simulink library "G2ELib_V1"  (R2020b)
settings: Solver=VariableStepAuto  StartTime=0.0  StopTime=10.0  RelTol=1e-3
undefined symbols (not defined in the file or in its folder): ee_sli_rtmsupport, Filter, Filter_I_ini, Filter_V_ini, gcbh, GFM, GFM_L2, GFM_R2, Parameters_Ib, Parameters_Sb, Parameters_Un_dc, q_filter_wf, References_Q, References_Theta_Eg0, simlt, sps_rtmsupport, Vdc_loop
libraries: powerlib x48, simulink_extras x11, eeTransforms x10, pid_lib x8, spsSourcesModel x3, powerlib_meascontrol x3, spsVIMeasurementModel x3, spsFirstOrderFilterModel x3, spsSynchronousMachineModel x3, eeGeneralControl x2, eePowerMeasurement x1, sps3phSaturableTransformerModel x1
(part 4 of 5)

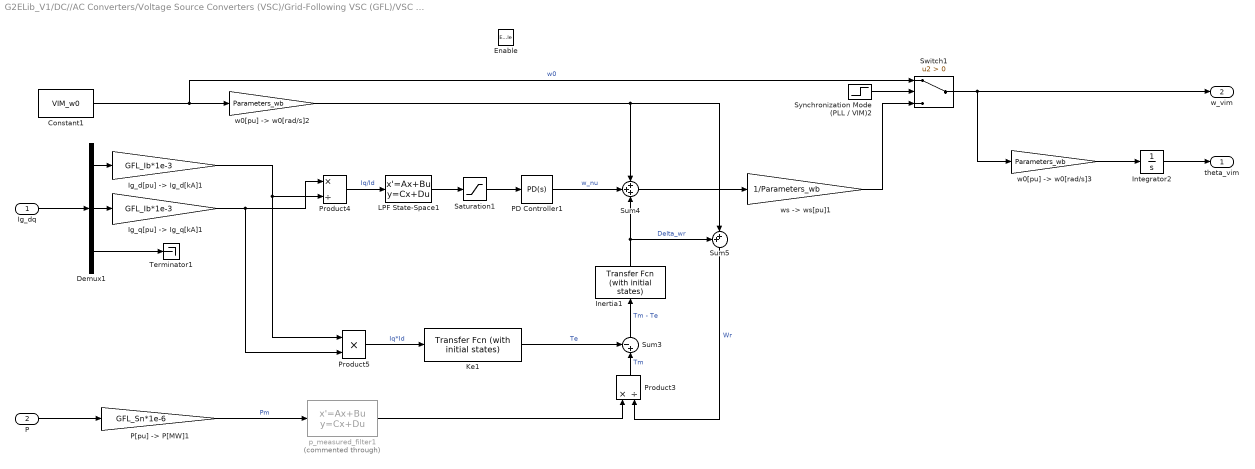
== system G2ELib_V1/DC//AC Converters/Voltage Source Converters (VSC)/Grid-Following VSC (GFL)/VSC - GFL - Ideal/VIM SU ==
  Ig_dq : Inport
  P : Inport  Port=2
  Enable : EnablePort
  Constant1 : Constant  Value=VIM_w0
  Demux1 : Demux  Outputs=3
      settings: DisplayOption=none
  "Ig_d[pu] -> Ig_d[kA]1" : Gain  Gain=GFL_Ib*1e-3
  "Ig_q[pu] -> Ig_q[kA]1" : Gain  Gain=GFL_Ib*1e-3
  Inertia1 : simulink_extras/Additional Linear/Transfer Fcn (with initial states)  N=1  D=[VIM_J VIM_D]  X0=VIM_Inertia_ini
  Integrator2 : Integrator  InitialCondition=GFL_theta
  Ke1 : simulink_extras/Additional Linear/Transfer Fcn (with initial states)  N=3/2.*VIM_Rr.*VIM_Lm.^2  D=[VIM_Lr.^2 , VIM_Rr.*VIM_Lr]  X0=VIM_Ke_ini
  LPF State-Space1 : StateSpace  A=-VIM_wc  C=VIM_wc  D=0  InitialCondition=VIM_wc_ini
  PD Controller1 : pid_lib/PID Controller  Controller=PD  Form=Parallel  TimeDomain=Continuous-time  UseExternalTs=off  SampleTime=-1  IntegratorMethod=Forward Euler  FilterMethod=Forward Euler  ControllerParametersSource=internal  P=VIM_Kp  I=0  D=VIM_Kd  UseFilter=on  N=VIM_Nd  TunerSelectOption=Transfer Function Based (PID Tuner App)  InitialConditionSource=internal  InitialConditionForIntegrator=0  InitialConditionForFilter=0  DifferentiatorICPrevScaledInput=0  ExternalReset=none  TrackingMode=off  Kt=1  LimitOutput=off  SatLimitsSource=internal  UpperSaturationLimit=inf  LowerSaturationLimit=-inf  LinearizeAsGain=on  AntiWindupMode=none  Kb=1  POutMin=[]  POutMax=[]  IOutMin=[]  IOutMax=[]  DOutMin=[]  DOutMax=[]  NOutMin=[]  NOutMax=[]  SumOutMin=[]  SumOutMax=[]  SaturationOutMin=[]  SaturationOutMax=[]  PParamMin=[]  PParamMax=[]  IParamMin=[]  IParamMax=[]  DParamMin=[]  DParamMax=[]  NParamMin=[]  NParamMax=[]  KbParamMin=[]  KbParamMax=[]  KtParamMin=[]  KtParamMax=[]  KbOutMin=[]  KbOutMax=[]  KtOutMin=[]  KtOutMax=[]  IntegratorOutMin=[]  IntegratorOutMax=[]  FilterOutMin=[]  FilterOutMax=[]  SumI1OutMin=[]  SumI1OutMax=[]  SumI2OutMin=[]  SumI2OutMax=[]  SumI3OutMin=[]  SumI3OutMax=[]  SumI4OutMin=[]  SumI4OutMax=[]  SumDOutMin=[]  SumDOutMax=[]  DifferentiatorOutMin=[]  DifferentiatorOutMax=[]  FilterDiffOutCoefMin=[]  FilterDiffOutCoefMax=[]  ReciprocalOutMin=[]  ReciprocalOutMax=[]  SumDenOutMin=[]  SumDenOutMax=[]  SumNumOutMin=[]  SumNumOutMax=[]  DivideOutMin=[]  DivideOutMax=[]  UdiffTsProdOutMin=[]  UdiffTsProdOutMax=[]  NTsProdOutMin=[]  NTsProdOutMax=[]  UintegralTsProdOutMin=[]  UintegralTsProdOutMax=[]  UngainTsProdOutMin=[]  UngainTsProdOutMax=[]  IntegratorContinuousStateAttributes=''  IntegratorStateMustResolveToSignalObject=off  IntegratorRTWStateStorageClass=Auto  FilterContinuousStateAttributes=''  FilterStateMustResolveToSignalObject=off  FilterRTWStateStorageClass=Auto  ParallelPVariant=InternalParameters  IdealPVariant=Disabled  IVariant=Disabled  DVariant=InternalParameters  IntegratorVariant=Disabled  SatVariant=Disabled  AWVariant=Disabled  PCopyVariant=Disabled  TRVariant=Disabled  FdbkBlocksVariant=Forward  IdealPFdbkVariant=Disabled  SatFdbkVariant=Disabled  DerivativeFilterVariant=ContFilter  NVariant=InternalParameters  NCopyVariant=Disabled  FilterICVariant=InternalICsFilter  IntegratorICVariant=Disabled  ExternalResetVariant=Disabled  TRSumVariant=Passthrough  SumFdbkVariant=Disabled  SumVariant=Sum_PD  TsampFilterVariant=InternalTs  TsampNgainVariant=Passthrough  TsampIntegralVariant=Disabled_SignalSpec  ExternalSaturationOutDataTypeStr=Inherit: Same as second input
  "P[pu] -> P[MW]1" : Gain  Gain=GFL_Sn*1e-6
  Product3 : Product  Inputs=*/
  Product4 : Product  Inputs=*/
  Product5 : Product
  Saturation1 : Saturate  UpperLimit=VIM_Iqd_sat  LowerLimit=-VIM_Iqd_sat
  Sum3 : Sum  Inputs=-+|
  Sum4 : Sum  Inputs=+++
  Sum5 : Sum  Inputs=++|
  Switch1 : Switch  Criteria=u2 > Threshold
  Synchronization Mode (PLL / VIM)2 : Step  Time=VIM_T_sync  Before=1  After=0  SampleTime=0
  Terminator1 : Terminator
  p_measured_filter1 : StateSpace  Commented=through  A=-q_filter_wf  C=q_filter_wf  D=0  InitialCondition=0
  "w0[pu] -> w0[rad/s]2" : Gain  Gain=Parameters_wb
  "w0[pu] -> w0[rad/s]3" : Gain  Gain=Parameters_wb
  "ws -> ws[pu]1" : Gain  Gain=1/Parameters_wb
  theta_vim : Outport
  w_vim : Outport  Port=2
  wires:
  p_measured_filter1/1 -> Product3/1
  Integrator2/1 -> theta_vim/1
  "w0[pu] -> w0[rad/s]3"/1 -> Integrator2/1
  Switch1/1 -> w_vim/1, "w0[pu] -> w0[rad/s]3"/1
  P/1 -> "P[pu] -> P[MW]1"/1
  Product4/1 -> LPF State-Space1/1  "Iq/Id"
  "Ig_q[pu] -> Ig_q[kA]1"/1 -> Product4/1, Product5/2
  Product3/1 -> Sum3/2  "Tm"
  PD Controller1/1 -> Sum4/2  "w_nu"
  Ke1/1 -> Sum3/1  "Te"
  Demux1/1 -> "Ig_d[pu] -> Ig_d[kA]1"/1
  Synchronization Mode (PLL / VIM)2/1 -> Switch1/2
  Sum4/1 -> "ws -> ws[pu]1"/1
  Demux1/2 -> "Ig_q[pu] -> Ig_q[kA]1"/1
  "Ig_d[pu] -> Ig_d[kA]1"/1 -> Product4/2, Product5/1
  Demux1/3 -> Terminator1/1
  Inertia1/1 -> Sum5/1, Sum4/3  "Delta_wr"
  Sum5/1 -> Product3/2  "Wr"
  LPF State-Space1/1 -> Saturation1/1
  Ig_dq/1 -> Demux1/1
  Product5/1 -> Ke1/1  "Iq*Id"
  Saturation1/1 -> PD Controller1/1
  "w0[pu] -> w0[rad/s]2"/1 -> Sum5/2, Sum4/1
  "P[pu] -> P[MW]1"/1 -> p_measured_filter1/1  "Pm"
  Sum3/1 -> Inertia1/1  "Tm - Te"
  "ws -> ws[pu]1"/1 -> Switch1/3
  Constant1/1 -> "w0[pu] -> w0[rad/s]2"/1, Switch1/1  "w0"

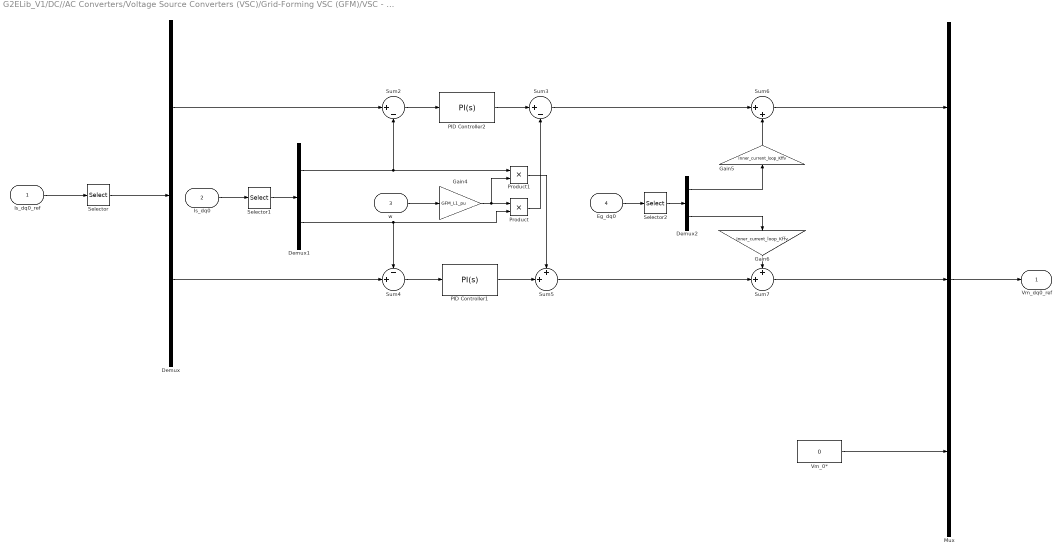
== system G2ELib_V1/DC//AC Converters/Voltage Source Converters (VSC)/Grid-Forming VSC (GFM)/VSC - GFM - Generic - Ideal/Current Loop ==
  Is_dq0_ref : Inport
  Is_dq0 : Inport  Port=2
  w : Inport  Port=3
  Eg_dq0 : Inport  Port=4
  Demux : Demux  Outputs=2
  Demux1 : Demux  Outputs=2
  Demux2 : Demux  Outputs=2
  Gain4 : Gain  Gain=GFM_L1_pu
  Gain5 : Gain  Gain=Inner_current_loop_Kffv
  Gain6 : Gain  Gain=Inner_current_loop_Kffv
  Mux : Mux  Inputs=3
  PID Controller1 : pid_lib/PID Controller  Controller=PI  Form=Parallel  TimeDomain=Continuous-time  UseExternalTs=off  SampleTime=-1  IntegratorMethod=Forward Euler  FilterMethod=Forward Euler  ControllerParametersSource=internal  P=Inner_current_loop_Kp  I=Inner_current_loop_Ki  D=0  UseFilter=on  N=100  TunerSelectOption=Transfer Function Based (PID Tuner App)  InitialConditionSource=internal  InitialConditionForIntegrator=Inner_current_loop_Int_ini_q  InitialConditionForFilter=0  DifferentiatorICPrevScaledInput=0  ExternalReset=none  TrackingMode=off  Kt=1  LimitOutput=off  SatLimitsSource=internal  UpperSaturationLimit=inf  LowerSaturationLimit=-inf  LinearizeAsGain=on  AntiWindupMode=none  Kb=1  POutMin=[]  POutMax=[]  IOutMin=[]  IOutMax=[]  DOutMin=[]  DOutMax=[]  NOutMin=[]  NOutMax=[]  SumOutMin=[]  SumOutMax=[]  SaturationOutMin=[]  SaturationOutMax=[]  PParamMin=[]  PParamMax=[]  IParamMin=[]  IParamMax=[]  DParamMin=[]  DParamMax=[]  NParamMin=[]  NParamMax=[]  KbParamMin=[]  KbParamMax=[]  KtParamMin=[]  KtParamMax=[]  KbOutMin=[]  KbOutMax=[]  KtOutMin=[]  KtOutMax=[]  IntegratorOutMin=[]  IntegratorOutMax=[]  FilterOutMin=[]  FilterOutMax=[]  SumI1OutMin=[]  SumI1OutMax=[]  SumI2OutMin=[]  SumI2OutMax=[]  SumI3OutMin=[]  SumI3OutMax=[]  SumI4OutMin=[]  SumI4OutMax=[]  SumDOutMin=[]  SumDOutMax=[]  DifferentiatorOutMin=[]  DifferentiatorOutMax=[]  FilterDiffOutCoefMin=[]  FilterDiffOutCoefMax=[]  ReciprocalOutMin=[]  ReciprocalOutMax=[]  SumDenOutMin=[]  SumDenOutMax=[]  SumNumOutMin=[]  SumNumOutMax=[]  DivideOutMin=[]  DivideOutMax=[]  UdiffTsProdOutMin=[]  UdiffTsProdOutMax=[]  NTsProdOutMin=[]  NTsProdOutMax=[]  UintegralTsProdOutMin=[]  UintegralTsProdOutMax=[]  UngainTsProdOutMin=[]  UngainTsProdOutMax=[]  IntegratorContinuousStateAttributes=''  IntegratorStateMustResolveToSignalObject=off  IntegratorRTWStateStorageClass=Auto  FilterContinuousStateAttributes=''  FilterStateMustResolveToSignalObject=off  FilterRTWStateStorageClass=Auto  ParallelPVariant=InternalParameters  IdealPVariant=Disabled  IVariant=InternalParameters  DVariant=Disabled  IntegratorVariant=Continuous  SatVariant=Disabled  AWVariant=Passthrough  PCopyVariant=Disabled  TRVariant=Disabled  FdbkBlocksVariant=Forward  IdealPFdbkVariant=Disabled  SatFdbkVariant=Disabled  DerivativeFilterVariant=Disabled  NVariant=Disabled  NCopyVariant=Disabled_SignalSpec  FilterICVariant=Disabled  IntegratorICVariant=InternalICs  ExternalResetVariant=Disabled  TRSumVariant=Passthrough  SumFdbkVariant=Disabled  SumVariant=Sum_PI  TsampFilterVariant=InternalTs  TsampNgainVariant=Passthrough  TsampIntegralVariant=Passthrough  ExternalSaturationOutDataTypeStr=Inherit: Same as second input
  PID Controller2 : pid_lib/PID Controller  Controller=PI  Form=Parallel  TimeDomain=Continuous-time  UseExternalTs=off  SampleTime=-1  IntegratorMethod=Forward Euler  FilterMethod=Forward Euler  ControllerParametersSource=internal  P=Inner_current_loop_Kp  I=Inner_current_loop_Ki  D=0  UseFilter=on  N=100  TunerSelectOption=Transfer Function Based (PID Tuner App)  InitialConditionSource=internal  InitialConditionForIntegrator=Inner_current_loop_Int_ini_d  InitialConditionForFilter=0  DifferentiatorICPrevScaledInput=0  ExternalReset=none  TrackingMode=off  Kt=1  LimitOutput=off  SatLimitsSource=internal  UpperSaturationLimit=inf  LowerSaturationLimit=-inf  LinearizeAsGain=on  AntiWindupMode=none  Kb=1  POutMin=[]  POutMax=[]  IOutMin=[]  IOutMax=[]  DOutMin=[]  DOutMax=[]  NOutMin=[]  NOutMax=[]  SumOutMin=[]  SumOutMax=[]  SaturationOutMin=[]  SaturationOutMax=[]  PParamMin=[]  PParamMax=[]  IParamMin=[]  IParamMax=[]  DParamMin=[]  DParamMax=[]  NParamMin=[]  NParamMax=[]  KbParamMin=[]  KbParamMax=[]  KtParamMin=[]  KtParamMax=[]  KbOutMin=[]  KbOutMax=[]  KtOutMin=[]  KtOutMax=[]  IntegratorOutMin=[]  IntegratorOutMax=[]  FilterOutMin=[]  FilterOutMax=[]  SumI1OutMin=[]  SumI1OutMax=[]  SumI2OutMin=[]  SumI2OutMax=[]  SumI3OutMin=[]  SumI3OutMax=[]  SumI4OutMin=[]  SumI4OutMax=[]  SumDOutMin=[]  SumDOutMax=[]  DifferentiatorOutMin=[]  DifferentiatorOutMax=[]  FilterDiffOutCoefMin=[]  FilterDiffOutCoefMax=[]  ReciprocalOutMin=[]  ReciprocalOutMax=[]  SumDenOutMin=[]  SumDenOutMax=[]  SumNumOutMin=[]  SumNumOutMax=[]  DivideOutMin=[]  DivideOutMax=[]  UdiffTsProdOutMin=[]  UdiffTsProdOutMax=[]  NTsProdOutMin=[]  NTsProdOutMax=[]  UintegralTsProdOutMin=[]  UintegralTsProdOutMax=[]  UngainTsProdOutMin=[]  UngainTsProdOutMax=[]  IntegratorContinuousStateAttributes=''  IntegratorStateMustResolveToSignalObject=off  IntegratorRTWStateStorageClass=Auto  FilterContinuousStateAttributes=''  FilterStateMustResolveToSignalObject=off  FilterRTWStateStorageClass=Auto  ParallelPVariant=InternalParameters  IdealPVariant=Disabled  IVariant=InternalParameters  DVariant=Disabled  IntegratorVariant=Continuous  SatVariant=Disabled  AWVariant=Passthrough  PCopyVariant=Disabled  TRVariant=Disabled  FdbkBlocksVariant=Forward  IdealPFdbkVariant=Disabled  SatFdbkVariant=Disabled  DerivativeFilterVariant=Disabled  NVariant=Disabled  NCopyVariant=Disabled_SignalSpec  FilterICVariant=Disabled  IntegratorICVariant=InternalICs  ExternalResetVariant=Disabled  TRSumVariant=Passthrough  SumFdbkVariant=Disabled  SumVariant=Sum_PI  TsampFilterVariant=InternalTs  TsampNgainVariant=Passthrough  TsampIntegralVariant=Passthrough  ExternalSaturationOutDataTypeStr=Inherit: Same as second input
  Product : Product
  Product1 : Product
  Selector : Selector  InputPortWidth=3  IndexOptions=Index vector (dialog)  Indices=[1 2]  OutputSizes=1
  Selector1 : Selector  InputPortWidth=3  IndexOptions=Index vector (dialog)  Indices=[1 2]  OutputSizes=1
  Selector2 : Selector  InputPortWidth=3  IndexOptions=Index vector (dialog)  Indices=[1 2]  OutputSizes=1
  Sum2 : Sum  Inputs=|+-
  Sum3 : Sum  Inputs=|+-
  Sum4 : Sum  Inputs=-+|
  Sum5 : Sum  Inputs=++|
  Sum6 : Sum  Inputs=|++
  Sum7 : Sum  Inputs=++|
  Vm_0* : Constant  Value=0
  Vm_dq0_ref : Outport
  wires:
  Demux1/1 -> Sum2/2, Product1/1
  Demux2/2 -> Gain6/1
  Demux2/1 -> Gain5/1
  Demux1/2 -> Sum4/1, Product/2
  PID Controller2/1 -> Sum3/1
  Selector/1 -> Demux/1
  Sum3/1 -> Sum6/1
  Gain5/1 -> Sum6/2
  Demux/1 -> Sum2/1
  PID Controller1/1 -> Sum5/2
  Gain4/1 -> Product1/2, Product/1
  Product/1 -> Sum3/2
  Selector1/1 -> Demux1/1
  w/1 -> Gain4/1
  Selector2/1 -> Demux2/1
  Vm_0*/1 -> Mux/3
  Is_dq0/1 -> Selector1/1
  Mux/1 -> Vm_dq0_ref/1
  Gain6/1 -> Sum7/1
  Sum2/1 -> PID Controller2/1
  Eg_dq0/1 -> Selector2/1
  Sum5/1 -> Sum7/2
  Sum4/1 -> PID Controller1/1
  Is_dq0_ref/1 -> Selector/1
  Product1/1 -> Sum5/1
  Demux/2 -> Sum4/2
  Sum6/1 -> Mux/1
  Sum7/1 -> Mux/2

== system G2ELib_V1/DC//AC Converters/Voltage Source Converters (VSC)/Grid-Forming VSC (GFM)/VSC - GFM - Generic - Ideal/DC Voltage Control  ==
  Vdc : Inport
  Vdc_ref : Inport  Port=2
  P_set : Inport  Port=3
  Gain : Gain  Gain=Vdc_loop_Ki
  Gain1 : Gain  Gain=Vdc_loop_Kp
  Gain2 : Gain  Gain=Parameters_Sb/(Parameters_Un_dc)
  Gain3 : Gain  Gain=Vdc_loop_Kffi
  Integrator : Integrator
  Sum : Sum  Inputs=|-+
  Sum1 : Sum  Inputs=+++
  idc_ref : Outport
  wires:
  Gain3/1 -> Sum1/1
  Gain2/1 -> Gain3/1
  Sum/1 -> Gain1/1, Gain/1
  Gain/1 -> Integrator/1
  P_set/1 -> Gain2/1
  Vdc/1 -> Sum/1
  Integrator/1 -> Sum1/2
  Sum1/1 -> idc_ref/1
  Vdc_ref/1 -> Sum/2
  Gain1/1 -> Sum1/3

== system G2ELib_V1/DC//AC Converters/Voltage Source Converters (VSC)/Grid-Forming VSC (GFM)/VSC - GFM - Generic - Ideal/Damping Resistor ==
  Ig_dq0 : Inport
  Gain : Gain  Gain=Damping_resistor_Rv
  Gain1 : Gain  Gain=Damping_resistor_Enable
  Subsystem : Subsystem
  Sum : Sum  Inputs=|+-
  dE_DR_dq0 : Outport
  wires:
  Gain1/1 -> dE_DR_dq0/1
  Sum/1 -> Gain1/1
  Subsystem/1(Out1) -> Sum/1
  Gain/1 -> Subsystem/1(In1), Sum/2
  Ig_dq0/1 -> Gain/1

== system G2ELib_V1/DC//AC Converters/Voltage Source Converters (VSC)/Grid-Forming VSC (GFM)/VSC - GFM - Generic - Ideal/Filter ==
  Ground : powerlib/Elements/Ground  LConnTagsString=a
  Series RLC Branch10 : PMComponent  DialogController=POWERSYS.PowerSysDialog  LoadFcn=sps_rtmsupport('LoadFcn',gcbh);  StartFcn=sps_rtmsupport('StartFcn',gcbh);  StopFcn=sps_rtmsupport('StopFcn',gcbh);  PhysicalDomain=powersysdomain  LeftPortType=p1  RightPortType=p1  LConnTagsString=__new0  RConnTagsString=__new0  mask(Series RLC Branch){BranchType=C, Resistance=GFM.R1, Inductance=GFM.L1, SetiL0=on, InitialCurrent=Filter.I_ini(1)*GFM.Ib, Capacitance=GFM_C, Setx0=off, InitialVoltage=Filter_V_ini(2), Measurements=None}
      mask prompts: BranchType "Branch type:"; Resistance "Resistance (Ohms):"; Inductance "Inductance (H):"; SetiL0 "Set the initial inductor current"; InitialCurrent "Inductor initial current (A):"; Capacitance "Capacitance (F):"; Setx0 "Set the initial capacitor voltage"; InitialVoltage "Capacitor initial voltage (V):"
      mask help:
      | Implements a series branch of RLC elements.
      | Use the 'Branch type' parameter to add or remove elements from the branch.
      mask init:
      | [s1,s2,s3,s4,r1,r2,l1,l2,c1,c2,c3,c4] = powericon('Series RLC Branch',Resistance,Inductance,Capacitance,BranchType);
      | powericon('RLCCback',gcb)
      | power_initmask();
      settings: CopyFcn=sps_rtmsupport('CopyFcn',gcbh);  DeleteFcn=sps_rtmsupport('DeleteFcn',gcbh);  UndoDeleteFcn=sps_rtmsupport('UndoDeleteFcn',gcbh);  ModelCloseFcn=sps_rtmsupport('ModelCloseFcn',gcbh);  PreSaveFcn=sps_rtmsupport('PreSaveFcn',gcbh);  PostSaveFcn=sps_rtmsupport('PostSaveFcn',gcbh);  NameChangeFcn=sps_rtmsupport('NameChangeFcn',gcbh);  PreCopyFcn=sps_rtmsupport('PreCopyFcn',gcbh);  OpenFcn=sps_rtmsupport('OpenFcn',gcbh, [1 4 7 9]);  CloseFcn=sps_rtmsupport('CloseFcn',gcbh);  PreDeleteFcn=sps_rtmsupport('PreDeleteFcn',gcbh);
      mask Help: helpview(psbhelp);
      mask TypeOptions BranchType: RLC | R | L | C | RL | RC | LC | Open circuit
      mask Callback BranchType: powericon('RLCCback',gcb)
      mask Callback Resistance: powericon('RLCCback',gcb)
      mask Callback Inductance: powericon('RLCCback',gcb)
      mask Callback SetiL0: powericon('RLCCback',gcb)
      mask Callback Capacitance: powericon('RLCCback',gcb)
      mask Callback Setx0: powericon('RLCCback',gcb)
      mask TypeOptions Measurements: None | Branch voltage | Branch current | Branch voltage and current
      mask Display:
      | plot(s1,s2,s3,s4,r1,r2*1.5,l1,l2*1.5,c1,c2*1.5,c3,c4*1.5)
      | color('red')
      | port_label('LConn',1,'+')
  Series RLC Branch11 : PMComponent  DialogController=POWERSYS.PowerSysDialog  LoadFcn=sps_rtmsupport('LoadFcn',gcbh);  StartFcn=sps_rtmsupport('StartFcn',gcbh);  StopFcn=sps_rtmsupport('StopFcn',gcbh);  PhysicalDomain=powersysdomain  LeftPortType=p1  RightPortType=p1  LConnTagsString=__new0  RConnTagsString=__new0  mask(Series RLC Branch){BranchType=C, Resistance=GFM.R1, Inductance=GFM.L1, SetiL0=on, InitialCurrent=Filter.I_ini(1)*GFM.Ib, Capacitance=GFM_C, Setx0=off, InitialVoltage=Filter_V_ini(3), Measurements=None}
      mask prompts: BranchType "Branch type:"; Resistance "Resistance (Ohms):"; Inductance "Inductance (H):"; SetiL0 "Set the initial inductor current"; InitialCurrent "Inductor initial current (A):"; Capacitance "Capacitance (F):"; Setx0 "Set the initial capacitor voltage"; InitialVoltage "Capacitor initial voltage (V):"
      mask help:
      | Implements a series branch of RLC elements.
      | Use the 'Branch type' parameter to add or remove elements from the branch.
      mask init:
      | [s1,s2,s3,s4,r1,r2,l1,l2,c1,c2,c3,c4] = powericon('Series RLC Branch',Resistance,Inductance,Capacitance,BranchType);
      | powericon('RLCCback',gcb)
      | power_initmask();
      settings: CopyFcn=sps_rtmsupport('CopyFcn',gcbh);  DeleteFcn=sps_rtmsupport('DeleteFcn',gcbh);  UndoDeleteFcn=sps_rtmsupport('UndoDeleteFcn',gcbh);  ModelCloseFcn=sps_rtmsupport('ModelCloseFcn',gcbh);  PreSaveFcn=sps_rtmsupport('PreSaveFcn',gcbh);  PostSaveFcn=sps_rtmsupport('PostSaveFcn',gcbh);  NameChangeFcn=sps_rtmsupport('NameChangeFcn',gcbh);  PreCopyFcn=sps_rtmsupport('PreCopyFcn',gcbh);  OpenFcn=sps_rtmsupport('OpenFcn',gcbh, [1 4 7 9]);  CloseFcn=sps_rtmsupport('CloseFcn',gcbh);  PreDeleteFcn=sps_rtmsupport('PreDeleteFcn',gcbh);
      mask Help: helpview(psbhelp);
      mask TypeOptions BranchType: RLC | R | L | C | RL | RC | LC | Open circuit
      mask Callback BranchType: powericon('RLCCback',gcb)
      mask Callback Resistance: powericon('RLCCback',gcb)
      mask Callback Inductance: powericon('RLCCback',gcb)
      mask Callback SetiL0: powericon('RLCCback',gcb)
      mask Callback Capacitance: powericon('RLCCback',gcb)
      mask Callback Setx0: powericon('RLCCback',gcb)
      mask TypeOptions Measurements: None | Branch voltage | Branch current | Branch voltage and current
      mask Display:
      | plot(s1,s2,s3,s4,r1,r2*1.5,l1,l2*1.5,c1,c2*1.5,c3,c4*1.5)
      | color('red')
      | port_label('LConn',1,'+')
  Series RLC Branch6 : PMComponent  DialogController=POWERSYS.PowerSysDialog  LoadFcn=sps_rtmsupport('LoadFcn',gcbh);  StartFcn=sps_rtmsupport('StartFcn',gcbh);  StopFcn=sps_rtmsupport('StopFcn',gcbh);  PhysicalDomain=powersysdomain  LeftPortType=p1  RightPortType=p1  LConnTagsString=__new0  RConnTagsString=__new0  mask(Series RLC Branch){BranchType=RL, Resistance=GFM_R1, Inductance=GFM_L1, SetiL0=off, InitialCurrent=Filter_I_ini(1), Capacitance=1e-6, Setx0=off, InitialVoltage=0, Measurements=None}
      mask prompts: BranchType "Branch type:"; Resistance "Resistance (Ohms):"; Inductance "Inductance (H):"; SetiL0 "Set the initial inductor current"; InitialCurrent "Inductor initial current (A):"; Capacitance "Capacitance (F):"; Setx0 "Set the initial capacitor voltage"; InitialVoltage "Capacitor initial voltage (V):"
      mask help:
      | Implements a series branch of RLC elements.
      | Use the 'Branch type' parameter to add or remove elements from the branch.
      mask init:
      | [s1,s2,s3,s4,r1,r2,l1,l2,c1,c2,c3,c4] = powericon('Series RLC Branch',Resistance,Inductance,Capacitance,BranchType);
      | powericon('RLCCback',gcb)
      | power_initmask();
      settings: CopyFcn=sps_rtmsupport('CopyFcn',gcbh);  DeleteFcn=sps_rtmsupport('DeleteFcn',gcbh);  UndoDeleteFcn=sps_rtmsupport('UndoDeleteFcn',gcbh);  ModelCloseFcn=sps_rtmsupport('ModelCloseFcn',gcbh);  PreSaveFcn=sps_rtmsupport('PreSaveFcn',gcbh);  PostSaveFcn=sps_rtmsupport('PostSaveFcn',gcbh);  NameChangeFcn=sps_rtmsupport('NameChangeFcn',gcbh);  PreCopyFcn=sps_rtmsupport('PreCopyFcn',gcbh);  OpenFcn=sps_rtmsupport('OpenFcn',gcbh, [1 4 7 9]);  CloseFcn=sps_rtmsupport('CloseFcn',gcbh);  PreDeleteFcn=sps_rtmsupport('PreDeleteFcn',gcbh);
      mask Help: helpview(psbhelp);
      mask TypeOptions BranchType: RLC | R | L | C | RL | RC | LC | Open circuit
      mask Callback BranchType: powericon('RLCCback',gcb)
      mask Callback Resistance: powericon('RLCCback',gcb)
      mask Callback Inductance: powericon('RLCCback',gcb)
      mask Callback SetiL0: powericon('RLCCback',gcb)
      mask Callback Capacitance: powericon('RLCCback',gcb)
      mask Callback Setx0: powericon('RLCCback',gcb)
      mask TypeOptions Measurements: None | Branch voltage | Branch current | Branch voltage and current
      mask Display:
      | plot(s1,s2,s3,s4,r1,r2*1.5,l1,l2*1.5,c1,c2*1.5,c3,c4*1.5)
      | color('red')
      | port_label('LConn',1,'+')
  Series RLC Branch7 : PMComponent  DialogController=POWERSYS.PowerSysDialog  LoadFcn=sps_rtmsupport('LoadFcn',gcbh);  StartFcn=sps_rtmsupport('StartFcn',gcbh);  StopFcn=sps_rtmsupport('StopFcn',gcbh);  PhysicalDomain=powersysdomain  LeftPortType=p1  RightPortType=p1  LConnTagsString=__new0  RConnTagsString=__new0  mask(Series RLC Branch){BranchType=RL, Resistance=GFM.R1, Inductance=GFM.L1, SetiL0=off, InitialCurrent=Filter_I_ini(2), Capacitance=1e-6, Setx0=off, InitialVoltage=0, Measurements=None}
      mask prompts: BranchType "Branch type:"; Resistance "Resistance (Ohms):"; Inductance "Inductance (H):"; SetiL0 "Set the initial inductor current"; InitialCurrent "Inductor initial current (A):"; Capacitance "Capacitance (F):"; Setx0 "Set the initial capacitor voltage"; InitialVoltage "Capacitor initial voltage (V):"
      mask help:
      | Implements a series branch of RLC elements.
      | Use the 'Branch type' parameter to add or remove elements from the branch.
      mask init:
      | [s1,s2,s3,s4,r1,r2,l1,l2,c1,c2,c3,c4] = powericon('Series RLC Branch',Resistance,Inductance,Capacitance,BranchType);
      | powericon('RLCCback',gcb)
      | power_initmask();
      settings: CopyFcn=sps_rtmsupport('CopyFcn',gcbh);  DeleteFcn=sps_rtmsupport('DeleteFcn',gcbh);  UndoDeleteFcn=sps_rtmsupport('UndoDeleteFcn',gcbh);  ModelCloseFcn=sps_rtmsupport('ModelCloseFcn',gcbh);  PreSaveFcn=sps_rtmsupport('PreSaveFcn',gcbh);  PostSaveFcn=sps_rtmsupport('PostSaveFcn',gcbh);  NameChangeFcn=sps_rtmsupport('NameChangeFcn',gcbh);  PreCopyFcn=sps_rtmsupport('PreCopyFcn',gcbh);  OpenFcn=sps_rtmsupport('OpenFcn',gcbh, [1 4 7 9]);  CloseFcn=sps_rtmsupport('CloseFcn',gcbh);  PreDeleteFcn=sps_rtmsupport('PreDeleteFcn',gcbh);
      mask Help: helpview(psbhelp);
      mask TypeOptions BranchType: RLC | R | L | C | RL | RC | LC | Open circuit
      mask Callback BranchType: powericon('RLCCback',gcb)
      mask Callback Resistance: powericon('RLCCback',gcb)
      mask Callback Inductance: powericon('RLCCback',gcb)
      mask Callback SetiL0: powericon('RLCCback',gcb)
      mask Callback Capacitance: powericon('RLCCback',gcb)
      mask Callback Setx0: powericon('RLCCback',gcb)
      mask TypeOptions Measurements: None | Branch voltage | Branch current | Branch voltage and current
      mask Display:
      | plot(s1,s2,s3,s4,r1,r2*1.5,l1,l2*1.5,c1,c2*1.5,c3,c4*1.5)
      | color('red')
      | port_label('LConn',1,'+')
  Series RLC Branch8 : PMComponent  DialogController=POWERSYS.PowerSysDialog  LoadFcn=sps_rtmsupport('LoadFcn',gcbh);  StartFcn=sps_rtmsupport('StartFcn',gcbh);  StopFcn=sps_rtmsupport('StopFcn',gcbh);  PhysicalDomain=powersysdomain  LeftPortType=p1  RightPortType=p1  LConnTagsString=__new0  RConnTagsString=__new0  mask(Series RLC Branch){BranchType=RL, Resistance=GFM.R1, Inductance=GFM.L1, SetiL0=off, InitialCurrent=Filter_I_ini(3), Capacitance=1e-6, Setx0=off, InitialVoltage=0, Measurements=None}
      mask prompts: BranchType "Branch type:"; Resistance "Resistance (Ohms):"; Inductance "Inductance (H):"; SetiL0 "Set the initial inductor current"; InitialCurrent "Inductor initial current (A):"; Capacitance "Capacitance (F):"; Setx0 "Set the initial capacitor voltage"; InitialVoltage "Capacitor initial voltage (V):"
      mask help:
      | Implements a series branch of RLC elements.
      | Use the 'Branch type' parameter to add or remove elements from the branch.
      mask init:
      | [s1,s2,s3,s4,r1,r2,l1,l2,c1,c2,c3,c4] = powericon('Series RLC Branch',Resistance,Inductance,Capacitance,BranchType);
      | powericon('RLCCback',gcb)
      | power_initmask();
      settings: CopyFcn=sps_rtmsupport('CopyFcn',gcbh);  DeleteFcn=sps_rtmsupport('DeleteFcn',gcbh);  UndoDeleteFcn=sps_rtmsupport('UndoDeleteFcn',gcbh);  ModelCloseFcn=sps_rtmsupport('ModelCloseFcn',gcbh);  PreSaveFcn=sps_rtmsupport('PreSaveFcn',gcbh);  PostSaveFcn=sps_rtmsupport('PostSaveFcn',gcbh);  NameChangeFcn=sps_rtmsupport('NameChangeFcn',gcbh);  PreCopyFcn=sps_rtmsupport('PreCopyFcn',gcbh);  OpenFcn=sps_rtmsupport('OpenFcn',gcbh, [1 4 7 9]);  CloseFcn=sps_rtmsupport('CloseFcn',gcbh);  PreDeleteFcn=sps_rtmsupport('PreDeleteFcn',gcbh);
      mask Help: helpview(psbhelp);
      mask TypeOptions BranchType: RLC | R | L | C | RL | RC | LC | Open circuit
      mask Callback BranchType: powericon('RLCCback',gcb)
      mask Callback Resistance: powericon('RLCCback',gcb)
      mask Callback Inductance: powericon('RLCCback',gcb)
      mask Callback SetiL0: powericon('RLCCback',gcb)
      mask Callback Capacitance: powericon('RLCCback',gcb)
      mask Callback Setx0: powericon('RLCCback',gcb)
      mask TypeOptions Measurements: None | Branch voltage | Branch current | Branch voltage and current
      mask Display:
      | plot(s1,s2,s3,s4,r1,r2*1.5,l1,l2*1.5,c1,c2*1.5,c3,c4*1.5)
      | color('red')
      | port_label('LConn',1,'+')
  Series RLC Branch9 : PMComponent  DialogController=POWERSYS.PowerSysDialog  LoadFcn=sps_rtmsupport('LoadFcn',gcbh);  StartFcn=sps_rtmsupport('StartFcn',gcbh);  StopFcn=sps_rtmsupport('StopFcn',gcbh);  PhysicalDomain=powersysdomain  LeftPortType=p1  RightPortType=p1  LConnTagsString=__new0  RConnTagsString=__new0  mask(Series RLC Branch){BranchType=C, Resistance=GFM.R1, Inductance=GFM.L1, SetiL0=on, InitialCurrent=Filter.I_ini(1)*GFM.Ib, Capacitance=GFM_C, Setx0=off, InitialVoltage=Filter_V_ini(1), Measurements=None}
      mask prompts: BranchType "Branch type:"; Resistance "Resistance (Ohms):"; Inductance "Inductance (H):"; SetiL0 "Set the initial inductor current"; InitialCurrent "Inductor initial current (A):"; Capacitance "Capacitance (F):"; Setx0 "Set the initial capacitor voltage"; InitialVoltage "Capacitor initial voltage (V):"
      mask help:
      | Implements a series branch of RLC elements.
      | Use the 'Branch type' parameter to add or remove elements from the branch.
      mask init:
      | [s1,s2,s3,s4,r1,r2,l1,l2,c1,c2,c3,c4] = powericon('Series RLC Branch',Resistance,Inductance,Capacitance,BranchType);
      | powericon('RLCCback',gcb)
      | power_initmask();
      settings: CopyFcn=sps_rtmsupport('CopyFcn',gcbh);  DeleteFcn=sps_rtmsupport('DeleteFcn',gcbh);  UndoDeleteFcn=sps_rtmsupport('UndoDeleteFcn',gcbh);  ModelCloseFcn=sps_rtmsupport('ModelCloseFcn',gcbh);  PreSaveFcn=sps_rtmsupport('PreSaveFcn',gcbh);  PostSaveFcn=sps_rtmsupport('PostSaveFcn',gcbh);  NameChangeFcn=sps_rtmsupport('NameChangeFcn',gcbh);  PreCopyFcn=sps_rtmsupport('PreCopyFcn',gcbh);  OpenFcn=sps_rtmsupport('OpenFcn',gcbh, [1 4 7 9]);  CloseFcn=sps_rtmsupport('CloseFcn',gcbh);  PreDeleteFcn=sps_rtmsupport('PreDeleteFcn',gcbh);
      mask Help: helpview(psbhelp);
      mask TypeOptions BranchType: RLC | R | L | C | RL | RC | LC | Open circuit
      mask Callback BranchType: powericon('RLCCback',gcb)
      mask Callback Resistance: powericon('RLCCback',gcb)
      mask Callback Inductance: powericon('RLCCback',gcb)
      mask Callback SetiL0: powericon('RLCCback',gcb)
      mask Callback Capacitance: powericon('RLCCback',gcb)
      mask Callback Setx0: powericon('RLCCback',gcb)
      mask TypeOptions Measurements: None | Branch voltage | Branch current | Branch voltage and current
      mask Display:
      | plot(s1,s2,s3,s4,r1,r2*1.5,l1,l2*1.5,c1,c2*1.5,c3,c4*1.5)
      | color('red')
      | port_label('LConn',1,'+')
  A : PMIOPort  Side=Left
  a : PMIOPort  Port=2  Side=Right
  B : PMIOPort  Port=3  Side=Left
  b : PMIOPort  Port=4  Side=Right
  C : PMIOPort  Port=5  Side=Left
  c : PMIOPort  Port=6  Side=Right
  connections:
  Series RLC Branch6/RConn1 -- a/RConn1 -- Series RLC Branch9/LConn1
  Series RLC Branch7/RConn1 -- b/RConn1 -- Series RLC Branch10/LConn1
  Series RLC Branch8/RConn1 -- c/RConn1 -- Series RLC Branch11/LConn1
  Series RLC Branch9/RConn1 -- Ground/LConn1 -- Series RLC Branch11/RConn1 -- Series RLC Branch10/RConn1
  C/RConn1 -- Series RLC Branch8/LConn1
  B/RConn1 -- Series RLC Branch7/LConn1
  A/RConn1 -- Series RLC Branch6/LConn1

== system G2ELib_V1/DC//AC Converters/Voltage Source Converters (VSC)/Grid-Forming VSC (GFM)/VSC - GFM - Generic - Ideal/Matching SU (SI) ==
  Vdc : Inport
  Vdc_ref : Inport  Port=2
  Enable : EnablePort
  Constant : Constant
  Gain : Gain  Gain=Matching_K_theta
  Gain1 : Gain
  Gain2 : Gain  Gain=1/GFM_Ub_dc
  Gain3 : Gain  Gain=Parameters_wb
  Gain4 : Gain
  Integrator : Integrator  InitialCondition=GFM_Theta_Eg0
  State-Space (with initial outputs)1 : simulink_extras/Additional Linear/State-Space (with initial outputs)  A=-q_filter_wf  B=1  C=q_filter_wf  D=0  U0=0  Y0=GFM_Vdcref/GFM_Ub_dc
      settings: SourceProductBaseCode=SL
  Sum : Sum  Inputs=|+-
  Sum1 : Sum  Inputs=++|
  theta : Outport
  w : Outport  Port=2
  wires:
  Gain/1 -> Sum1/2
  Vdc/1 -> Gain2/1
  Constant/1 -> Sum1/1
  Vdc_ref/1 -> Gain1/1
  Sum1/1 -> Gain4/1, Gain3/1
  Sum/1 -> Gain/1
  Integrator/1 -> theta/1
  Gain3/1 -> Integrator/1
  Gain1/1 -> Sum/2
  Gain4/1 -> w/1
  Gain2/1 -> State-Space (with initial outputs)1/1
  State-Space (with initial outputs)1/1 -> Sum/1

== system G2ELib_V1/DC//AC Converters/Voltage Source Converters (VSC)/Grid-Forming VSC (GFM)/VSC - GFM - Generic - Ideal/P-f Droop SU (PU) ==
  P : Inport
  P_set : Inport  Port=2
  w_set : Inport  Port=3
  Enable : EnablePort
  Gain : Gain  Gain=Droop_mp
  Gain1 : Gain  Gain=Parameters_wb
  Integrator : Integrator  InitialCondition=GFM_theta
  State-Space (with initial outputs) : simulink_extras/Additional Linear/State-Space (with initial outputs)  Commented=through  A=-Droop_wc  B=1  C=Droop_wc  D=0  U0=0  Y0=0
      settings: SourceProductBaseCode=SL
  State-Space (with initial outputs)1 : simulink_extras/Additional Linear/State-Space (with initial outputs)  A=-q_filter_wf  B=1  C=q_filter_wf  D=0  U0=0  Y0=GFM_Pref
      settings: SourceProductBaseCode=SL
  Sum : Sum  Inputs=+-|
  Sum1 : Sum  Inputs=++|
  theta : Outport
  w : Outport  Port=2
  wires:
  P/1 -> State-Space (with initial outputs)1/1
  Integrator/1 -> theta/1
  Gain1/1 -> Integrator/1
  Sum1/1 -> w/1, Gain1/1
  w_set/1 -> Sum1/1
  Sum/1 -> Gain/1
  Gain/1 -> State-Space (with initial outputs)/1
  P_set/1 -> Sum/1
  State-Space (with initial outputs)/1 -> Sum1/2
  State-Space (with initial outputs)1/1 -> Sum/2

== system G2ELib_V1/DC//AC Converters/Voltage Source Converters (VSC)/Grid-Forming VSC (GFM)/VSC - GFM - Generic - Ideal/PI_dc_voltage controller ==
  In : Inport
  Gain21 : Gain  Gain=Vdc_loop.Ki
  Gain22 : Gain  Gain=Vdc_loop.Kp
  Integrator1 : Integrator
  Sum6 : Sum  Inputs=++|
  out : Outport
  wires:
  Gain22/1 -> Sum6/1
  Integrator1/1 -> Sum6/2
  Gain21/1 -> Integrator1/1
  Sum6/1 -> out/1
  In/1 -> Gain21/1, Gain22/1

== system G2ELib_V1/DC//AC Converters/Voltage Source Converters (VSC)/Grid-Forming VSC (GFM)/VSC - GFM - Generic - Ideal/PLL ==
  Eg_abc : Inport
  Enable : EnablePort
  Constant : Constant
  Constant1 : Constant  Value=0
  Demux5 : Demux  Outputs=3
  Gain1 : Gain  Gain=0.0382
  Gain2 : Gain  Gain=0.2293
  Gain4 : Gain  Gain=Parameters_wb
  Integrator1 : Integrator  InitialCondition=GFM_theta
  Integrator3 : Integrator
  Low-Pass Filter (Discrete or Continuous) : eeGeneralControl/Low-Pass Filter (Discrete or Continuous)  Commented=through  K=1  T=0.01  B=inf  A=-inf  init_option=Specify as parameter  x0=1  Ts=simlt.T_step
  Park Transform3 : eeTransforms/Park Transform  AxisAlignment=Q-axis  PowerInvariant=off
  Sum : Sum  Inputs=|+-
  Sum1 : Sum  Inputs=|++
  Sum7 : Sum  Inputs=|++
  Terminator3 : Terminator
  Terminator4 : Terminator
  Transport Delay6 : TransportDelay  DelayTime=simlt.T_step  InitialOutput=Eg0_dq0
  w : Outport
  theta : Outport  Port=2
  wires:
  Sum7/1 -> Gain4/1, Low-Pass Filter (Discrete or Continuous)/1
  Gain2/1 -> Integrator3/1
  Gain4/1 -> Integrator1/1
  Eg_abc/1 -> Park Transform3/1
  Gain1/1 -> Sum1/1
  Demux5/2 -> Sum/1
  Sum1/1 -> Sum7/1
  Sum/1 -> Gain2/1, Gain1/1
  Demux5/3 -> Terminator3/1
  Demux5/1 -> Terminator4/1
  Integrator1/1 -> theta/1, Park Transform3/2
  Constant/1 -> Sum7/2
  Transport Delay6/1 -> Demux5/1
  Park Transform3/1 -> Transport Delay6/1
  Integrator3/1 -> Sum1/2
  Low-Pass Filter (Discrete or Continuous)/1 -> w/1
  Constant1/1 -> Sum/2

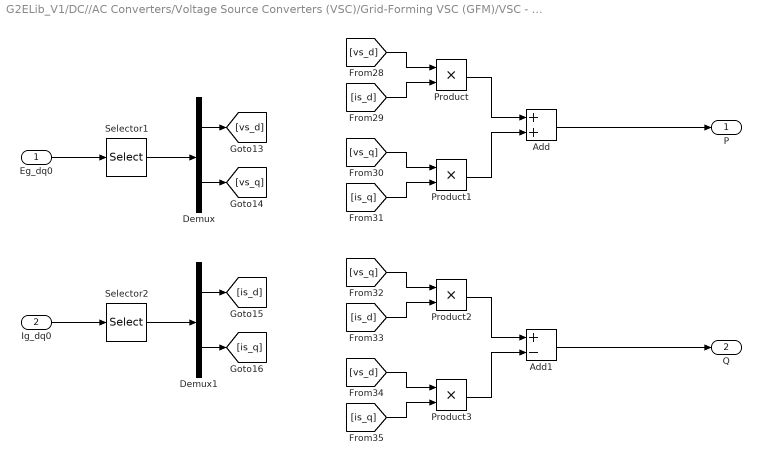
== system G2ELib_V1/DC//AC Converters/Voltage Source Converters (VSC)/Grid-Forming VSC (GFM)/VSC - GFM - Generic - Ideal/Power Measurement ==
  Eg_dq0 : Inport
  Ig_dq0 : Inport  Port=2
  Add : Sum
  Add1 : Sum  Inputs=+-
  Demux : Demux  Outputs=2
  Demux1 : Demux  Outputs=2
  Product{,1..3} (4 alike) : Product
  Selector1 : Selector  InputPortWidth=3  IndexOptions=Index vector (dialog)  Indices=[1 2]  OutputSizes=1
  Selector2 : Selector  InputPortWidth=3  IndexOptions=Index vector (dialog)  Indices=[1 2]  OutputSizes=1
  P : Outport
  Q : Outport  Port=2
  wires:
  Product/1 -> Add/1
  Product3/1 -> Add1/2
  Demux/1 -> [vs_d]
  [is_q] -> Product1/2
  [vs_q] -> Product1/1
  Selector2/1 -> Demux1/1
  [is_d] -> Product2/2
  [vs_d] -> Product3/1
  Product2/1 -> Add1/1
  Demux1/1 -> [is_d]
  [is_d] -> Product/2
  [vs_q] -> Product2/1
  Add1/1 -> Q/1
  Product1/1 -> Add/2
  [is_q] -> Product3/2
  Demux1/2 -> [is_q]
  Add/1 -> P/1
  Demux/2 -> [vs_q]
  [vs_d] -> Product/1
  Selector1/1 -> Demux/1
  Eg_dq0/1 -> Selector1/1
  Ig_dq0/1 -> Selector2/1

== system G2ELib_V1/DC//AC Converters/Voltage Source Converters (VSC)/Grid-Forming VSC (GFM)/VSC - GFM - Generic - Ideal/Q-V Droop MMU (PU) ==
  note: Generally only we set Eg_set_d only and Eg_set_q and Eg_set_0 equal zeros
  Q : Inport
  Q_set : Inport  Port=2
  Eg_set_dq0 : Inport  Port=3
  Enable : EnablePort
  Demux : Demux  Outputs=2
  Gain : Gain  Gain=Droop_nq
  Hypot : Math  Operator=hypot  SaturateOnIntegerOverflow=on
  Product : Product  Inputs=*/*
  Selector : Selector  InputPortWidth=3  IndexOptions=Index vector (dialog)  Indices=[1 2]  OutputSizes=1
  State-Space (with initial outputs)1 : simulink_extras/Additional Linear/State-Space (with initial outputs)  A=-q_filter_wf  B=1  C=q_filter_wf  D=0  U0=0  Y0=GFM_Qref
      settings: SourceProductBaseCode=SL
  Sum : Sum  Inputs=+-|
  Sum1 : Sum  Inputs=++|
  Eg_dq0_ref : Outport
  wires:
  Q/1 -> State-Space (with initial outputs)1/1
  Gain/1 -> Sum1/2
  Sum1/1 -> Product/1
  Q_set/1 -> Sum/1
  Eg_set_dq0/1 -> Product/3, Selector/1
  Selector/1 -> Demux/1
  Demux/2 -> Hypot/2
  Sum/1 -> Gain/1
  Demux/1 -> Hypot/1
  Hypot/1 -> Product/2, Sum1/1
  Product/1 -> Eg_dq0_ref/1
  State-Space (with initial outputs)1/1 -> Sum/2

== system G2ELib_V1/DC//AC Converters/Voltage Source Converters (VSC)/Grid-Forming VSC (GFM)/VSC - GFM - Generic - Ideal/Subsystem ==
  Vdq0 : Inport
  Add : Sum  Inputs=+++
  Demux : Demux  Outputs=3
  Product : Product
  Product1 : Product
  Product2 : Product
  Sqrt : Sqrt  SaturateOnIntegerOverflow=on
  Vrms : Outport
  wires:
  Add/1 -> Sqrt/1
  Product1/1 -> Add/2
  Sqrt/1 -> Vrms/1
  Vdq0/1 -> Demux/1
  Demux/2 -> Product1/1, Product1/2
  Product/1 -> Add/1
  Demux/1 -> Product/1, Product/2
  Demux/3 -> Product2/1, Product2/2
  Product2/1 -> Add/3

== system G2ELib_V1/DC//AC Converters/Voltage Source Converters (VSC)/Grid-Forming VSC (GFM)/VSC - GFM - Generic - Ideal/Subsystem1 ==
  Idq0 : Inport
  Add : Sum  Inputs=+++
  Demux : Demux  Outputs=3
  Product : Product
  Product1 : Product
  Product2 : Product
  Sqrt : Sqrt  SaturateOnIntegerOverflow=on
  Irms : Outport
  wires:
  Add/1 -> Sqrt/1
  Product1/1 -> Add/2
  Sqrt/1 -> Irms/1
  Idq0/1 -> Demux/1
  Demux/2 -> Product1/1, Product1/2
  Product/1 -> Add/1
  Demux/1 -> Product/1, Product/2
  Demux/3 -> Product2/1, Product2/2
  Product2/1 -> Add/3

== system G2ELib_V1/DC//AC Converters/Voltage Source Converters (VSC)/Grid-Forming VSC (GFM)/VSC - GFM - Generic - Ideal/Transient Virtual Impedance ==
  note: TVI triggering
  isd_mes_pu : Inport
  Demux : Demux  Outputs=2
  Demux1 : Demux  Outputs=2
      settings: DisplayOption=none
  Gain : Gain  Gain=TVI_K_RV
  Gain5 : Gain  Gain=TVI_Rho_XR
  Gain9 : Gain  Gain=TVI_Rho_XR
  Hypot : Math  Operator=hypot  SaturateOnIntegerOverflow=on
  I_tresh : Constant  Value=TVI_I_thresh_pu
  Mux2 : Mux  Inputs=3
  Selector1 : Selector  InputPortWidth=3  IndexOptions=Index vector (dialog)  Indices=[1 2]  OutputSizes=1
  Sum1 : Sum  Inputs=|+-
  Sum7 : Sum  Inputs=|+-
  Sum8 : Sum  Inputs=++|
  Switch2 : Switch
  dEg_0 : Constant  Value=0
  disabled : Constant  Value=0
  product{,1..3} (4 alike) : Product  InputSameDT=on  RndMeth=Zero  SaturateOnIntegerOverflow=on  OutDataTypeStr=Inherit: Same as first input
  dEg_dq0_VI : Outport
  wires:
  Gain9/1 -> Sum8/1
  I_tresh/1 -> Sum1/2
  Selector1/1 -> Switch2/1, Demux/1
  disabled/1 -> Switch2/3
  Switch2/1 -> Demux1/1
  Gain5/1 -> Sum7/2
  Sum1/1 -> Switch2/2, Gain/1
  dEg_0/1 -> Mux2/3
  product2/1 -> Sum8/2
  Demux/2 -> Hypot/2
  Demux/1 -> Hypot/1
  Demux1/2 -> product3/1, product2/1  "igq"
  isd_mes_pu/1 -> Selector1/1
  Demux1/1 -> product/2, product1/1  "Igd"
  Gain/1 -> product2/2, product1/2, product/1, product3/2
  Sum7/1 -> Mux2/1
  product3/1 -> Gain5/1
  product1/1 -> Sum7/1
  product/1 -> Gain9/1
  Sum8/1 -> Mux2/2
  Hypot/1 -> Sum1/1
  Mux2/1 -> dEg_dq0_VI/1

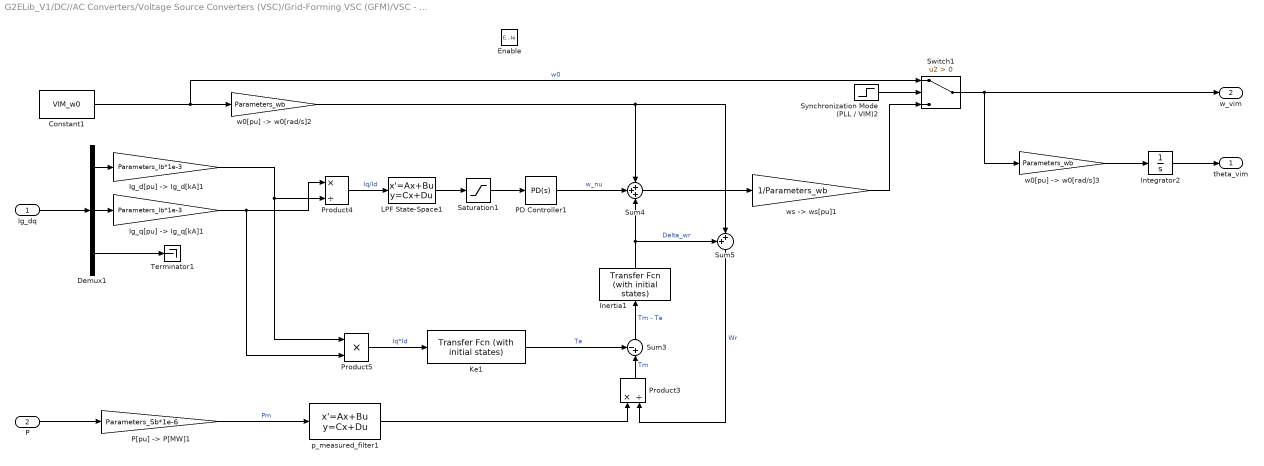
== system G2ELib_V1/DC//AC Converters/Voltage Source Converters (VSC)/Grid-Forming VSC (GFM)/VSC - GFM - Generic - Ideal/VIM SU ==
  Ig_dq : Inport
  P : Inport  Port=2
  Enable : EnablePort
  Constant1 : Constant  Value=VIM_w0
  Demux1 : Demux  Outputs=3
      settings: DisplayOption=none
  "Ig_d[pu] -> Ig_d[kA]1" : Gain  Gain=Parameters_Ib*1e-3
  "Ig_q[pu] -> Ig_q[kA]1" : Gain  Gain=Parameters_Ib*1e-3
  Inertia1 : simulink_extras/Additional Linear/Transfer Fcn (with initial states)  N=1  D=[VIM_J VIM_D]  X0=VIM_Inertia_ini
  Integrator2 : Integrator  InitialCondition=References_Theta_Eg0
  Ke1 : simulink_extras/Additional Linear/Transfer Fcn (with initial states)  N=3/2.*VIM_Rr.*VIM_Lm.^2  D=[VIM_Lr.^2 , VIM_Rr.*VIM_Lr]  X0=VIM_Ke_ini
  LPF State-Space1 : StateSpace  A=-VIM_wc  C=VIM_wc  D=0  InitialCondition=VIM_wc_ini
  PD Controller1 : pid_lib/PID Controller  Controller=PD  Form=Parallel  TimeDomain=Continuous-time  UseExternalTs=off  SampleTime=-1  IntegratorMethod=Forward Euler  FilterMethod=Forward Euler  ControllerParametersSource=internal  P=VIM_Kp  I=0  D=VIM_Kd  UseFilter=on  N=VIM_Nd  TunerSelectOption=Transfer Function Based (PID Tuner App)  InitialConditionSource=internal  InitialConditionForIntegrator=0  InitialConditionForFilter=0  DifferentiatorICPrevScaledInput=0  ExternalReset=none  TrackingMode=off  Kt=1  LimitOutput=off  SatLimitsSource=internal  UpperSaturationLimit=inf  LowerSaturationLimit=-inf  LinearizeAsGain=on  AntiWindupMode=none  Kb=1  POutMin=[]  POutMax=[]  IOutMin=[]  IOutMax=[]  DOutMin=[]  DOutMax=[]  NOutMin=[]  NOutMax=[]  SumOutMin=[]  SumOutMax=[]  SaturationOutMin=[]  SaturationOutMax=[]  PParamMin=[]  PParamMax=[]  IParamMin=[]  IParamMax=[]  DParamMin=[]  DParamMax=[]  NParamMin=[]  NParamMax=[]  KbParamMin=[]  KbParamMax=[]  KtParamMin=[]  KtParamMax=[]  KbOutMin=[]  KbOutMax=[]  KtOutMin=[]  KtOutMax=[]  IntegratorOutMin=[]  IntegratorOutMax=[]  FilterOutMin=[]  FilterOutMax=[]  SumI1OutMin=[]  SumI1OutMax=[]  SumI2OutMin=[]  SumI2OutMax=[]  SumI3OutMin=[]  SumI3OutMax=[]  SumI4OutMin=[]  SumI4OutMax=[]  SumDOutMin=[]  SumDOutMax=[]  DifferentiatorOutMin=[]  DifferentiatorOutMax=[]  FilterDiffOutCoefMin=[]  FilterDiffOutCoefMax=[]  ReciprocalOutMin=[]  ReciprocalOutMax=[]  SumDenOutMin=[]  SumDenOutMax=[]  SumNumOutMin=[]  SumNumOutMax=[]  DivideOutMin=[]  DivideOutMax=[]  UdiffTsProdOutMin=[]  UdiffTsProdOutMax=[]  NTsProdOutMin=[]  NTsProdOutMax=[]  UintegralTsProdOutMin=[]  UintegralTsProdOutMax=[]  UngainTsProdOutMin=[]  UngainTsProdOutMax=[]  IntegratorContinuousStateAttributes=''  IntegratorStateMustResolveToSignalObject=off  IntegratorRTWStateStorageClass=Auto  FilterContinuousStateAttributes=''  FilterStateMustResolveToSignalObject=off  FilterRTWStateStorageClass=Auto  ParallelPVariant=InternalParameters  IdealPVariant=Disabled  IVariant=Disabled  DVariant=InternalParameters  IntegratorVariant=Disabled  SatVariant=Disabled  AWVariant=Disabled  PCopyVariant=Disabled  TRVariant=Disabled  FdbkBlocksVariant=Forward  IdealPFdbkVariant=Disabled  SatFdbkVariant=Disabled  DerivativeFilterVariant=ContFilter  NVariant=InternalParameters  NCopyVariant=Disabled  FilterICVariant=InternalICsFilter  IntegratorICVariant=Disabled  ExternalResetVariant=Disabled  TRSumVariant=Passthrough  SumFdbkVariant=Disabled  SumVariant=Sum_PD  TsampFilterVariant=InternalTs  TsampNgainVariant=Passthrough  TsampIntegralVariant=Disabled_SignalSpec  ExternalSaturationOutDataTypeStr=Inherit: Same as second input
  "P[pu] -> P[MW]1" : Gain  Gain=Parameters_Sb*1e-6
  Product3 : Product  Inputs=*/
  Product4 : Product  Inputs=*/
  Product5 : Product
  Saturation1 : Saturate  UpperLimit=VIM_Iqd_sat  LowerLimit=-VIM_Iqd_sat
  Sum3 : Sum  Inputs=-+|
  Sum4 : Sum  Inputs=+++
  Sum5 : Sum  Inputs=++|
  Switch1 : Switch  Criteria=u2 > Threshold
  Synchronization Mode (PLL / VIM)2 : Step  Time=VIM_T_sync  Before=1  After=0  SampleTime=0
  Terminator1 : Terminator
  p_measured_filter1 : StateSpace  A=-q_filter_wf  C=q_filter_wf  D=0  InitialCondition=0
  "w0[pu] -> w0[rad/s]2" : Gain  Gain=Parameters_wb
  "w0[pu] -> w0[rad/s]3" : Gain  Gain=Parameters_wb
  "ws -> ws[pu]1" : Gain  Gain=1/Parameters_wb
  theta_vim : Outport
  w_vim : Outport  Port=2
  wires:
  p_measured_filter1/1 -> Product3/1
  Integrator2/1 -> theta_vim/1
  "w0[pu] -> w0[rad/s]3"/1 -> Integrator2/1
  Switch1/1 -> w_vim/1, "w0[pu] -> w0[rad/s]3"/1
  P/1 -> "P[pu] -> P[MW]1"/1
  Product4/1 -> LPF State-Space1/1  "Iq/Id"
  "Ig_q[pu] -> Ig_q[kA]1"/1 -> Product4/1, Product5/2
  Product3/1 -> Sum3/2  "Tm"
  PD Controller1/1 -> Sum4/2  "w_nu"
  Ke1/1 -> Sum3/1  "Te"
  Demux1/1 -> "Ig_d[pu] -> Ig_d[kA]1"/1
  Synchronization Mode (PLL / VIM)2/1 -> Switch1/2
  Sum4/1 -> "ws -> ws[pu]1"/1
  Demux1/2 -> "Ig_q[pu] -> Ig_q[kA]1"/1
  "Ig_d[pu] -> Ig_d[kA]1"/1 -> Product4/2, Product5/1
  Demux1/3 -> Terminator1/1
  Inertia1/1 -> Sum5/1, Sum4/3  "Delta_wr"
  Sum5/1 -> Product3/2  "Wr"
  LPF State-Space1/1 -> Saturation1/1
  Ig_dq/1 -> Demux1/1
  Product5/1 -> Ke1/1  "Iq*Id"
  Saturation1/1 -> PD Controller1/1
  "w0[pu] -> w0[rad/s]2"/1 -> Sum5/2, Sum4/1
  "P[pu] -> P[MW]1"/1 -> p_measured_filter1/1  "Pm"
  Sum3/1 -> Inertia1/1  "Tm - Te"
  "ws -> ws[pu]1"/1 -> Switch1/3
  Constant1/1 -> "w0[pu] -> w0[rad/s]2"/1, Switch1/1  "w0"

== system G2ELib_V1/DC//AC Converters/Voltage Source Converters (VSC)/Grid-Forming VSC (GFM)/VSC - GFM - Generic - Ideal/VSM AVR (PU) ==
  Eg_dq0_set : Inport
  Eg_dq0_pu : Inport  Port=2
  theta : Inport  Port=3
  w : Inport  Port=4
  Q_set : Inport  Port=5
  Q : Inport  Port=6
  Enable : EnablePort
  Demux : Demux  Outputs=2
  Demux1 : Demux  Outputs=3
  Demux2 : Demux  Commented=on  Outputs=3
  Gain : Gain  Gain=VSM_Dq
  Gain6 : Gain  Gain=1/VSM_K
  Hypot : Math  Operator=hypot  SaturateOnIntegerOverflow=on
  Integrator : Integrator  InitialCondition=1
  Mux : Mux  Inputs=3
  Park Transform2 : Subsystem  Commented=on  LoadFcn=ee_sli_rtmsupport( 'loadfcn', gcbh );  mask(Park Transform){AxisAlignment=Q-axis, PowerInvariant=off}
      mask prompts: AxisAlignment "physmod:ee:library:comments:control:eeTransforms:PhaseaAxisAlignment_MP"; PowerInvariant "physmod:ee:library:comments:control:eeTransforms:PowerInvariant_MP"
      mask help: physmod:ee:library:comments:control:eeTransforms:ParkTransform_MD
      mask init:
      | if PowerInvariant==0
      |     K1 = 0.5;
      |     K2 = 2/3;
      | else
      |     K1 = 1/sqrt(2);
      |     K2 = sqrt(2/3);
      | end
      | 
      | switch AxisAlignment
      |     case 'Q-axis'
      |         Offset = 0;
      |     case 'D-axis'
      |         Offset = pi/2;
      |     otherwise
      | end
      settings: CopyFcn=ee_sli_rtmsupport( 'copyfcn', gcbh );  DeleteFcn=ee_sli_rtmsupport( 'deletefcn', gcbh );  ModelCloseFcn=ee_sli_rtmsupport( 'modelclosefcn', gcbh );  PostSaveFcn=ee_sli_rtmsupport( 'postsavefcn', gcbh );  PreCopyFcn=ee_sli_rtmsupport( 'precopyfcn', gcbh );  OpenFcn=ee_sli_rtmsupport( 'openfcn', gcbh );  CloseFcn=ee_sli_rtmsupport( 'closefcn', gcbh );  PreDeleteFcn=ee_sli_rtmsupport( 'predeletefcn', gcbh );
      mask Help: web(nesl_help(gcbh))
      mask TypeOptions AxisAlignment: physmod:ee:library:comments:control:eeTransforms:Q0x2DAxis_PV | physmod:ee:library:comments:control:eeTransforms:D0x2DAxis_PV
      mask DialogControl AxisAlignment Prompt: Phase-a axis alignment
      mask DialogControl PowerInvariant Prompt: Power invariant
      mask Display: ee.mask.drawParkTransform();
  Product : Product
  Selector : Selector  InputPortWidth=3  IndexOptions=Index vector (dialog)  Indices=[1 2]  OutputSizes=1
  Sum : Sum  Inputs=-+|
  Sum1 : Sum  Inputs=++-
  Terminator : Terminator
  Terminator1 : Terminator
  Zero : Constant  Value=0  OutDataTypeStr=Inherit: Inherit via back propagation
  emf_ calculation2 : Subsystem  Commented=on
  Eg_dq0_ref : Outport
  wires:
  Q/1 -> Sum1/3
  Eg_dq0_set/1 -> Selector/1
  Demux1/3 -> Terminator1/1
  Sum1/1 -> Gain6/1
  Q_set/1 -> Sum1/2
  Gain/1 -> Sum1/1
  Demux/2 -> Hypot/2
  Demux/1 -> Hypot/1
  Hypot/1 -> Sum/2
  Selector/1 -> Demux/1
  Demux1/2 -> Terminator/1
  Gain6/1 -> Integrator/1
  Sum/1 -> Gain/1
  Eg_dq0_pu/1 -> Demux1/1
  Mux/1 -> Eg_dq0_ref/1
  Zero/1 -> Mux/3, Mux/2
  theta/1 -> ?
  ? -> emf_ calculation2/3(w)
  ? -> emf_ calculation2/1(MfIf)
  emf_ calculation2/1(emf) -> Park Transform2/1(abc)
  Demux2/2 -> ?
  Demux2/3 -> ?
  Demux2/1 -> ?
  Park Transform2/1(dq0) -> Demux2/1
  ? -> emf_ calculation2/2(theta)
  ? -> Park Transform2/2(theta)
  Integrator/1 -> Product/1
  w/1 -> Product/2
  Product/1 -> Mux/1, Sum/1

== system G2ELib_V1/DC//AC Converters/Voltage Source Converters (VSC)/Grid-Forming VSC (GFM)/VSC - GFM - Generic - Ideal/VSM SU (PU) ==
  P : Inport
  PA_set : Inport  Port=2
  w_set : Inport  Port=3
  Enable : EnablePort
  Gain1 : Gain  Commented=through  Gain=Parameters_wb
  Gain2 : Gain  Commented=through  Gain=GFM_Sn/Parameters_wb
  Gain3 : Gain  Commented=through  Gain=GFM_Sn/Parameters_wb
  Gain4 : Gain  Gain=Parameters_wb
  Gain5 : Gain  Gain=VSM_D
  Gain6 : Gain  Gain=1/VSM_J
  Gain7 : Gain  Commented=through  Gain=1/Parameters_wb
  Integrator : Integrator
  Integrator2 : Integrator  InitialCondition=GFM_Theta_Eg0
  Sum : Sum  Inputs=-|+|-
  Sum1 : Sum  Inputs=+|+||
  theta : Outport  VectorParamsAs1DForOutWhenUnconnected=off
  w : Outport  Port=2  VectorParamsAs1DForOutWhenUnconnected=off
  wires:
  Gain1/1 -> Sum1/1
  Gain6/1 -> Integrator/1
  Gain7/1 -> w/1
  Gain4/1 -> Integrator2/1
  Sum1/1 -> Gain7/1, Gain4/1
  Integrator2/1 -> theta/1
  P/1 -> Gain3/1
  Gain3/1 -> Sum/3
  PA_set/1 -> Gain2/1
  w_set/1 -> Gain1/1
  Integrator/1 -> Sum1/2, Gain5/1
  Gain5/1 -> Sum/1
  Sum/1 -> Gain6/1
  Gain2/1 -> Sum/2

== system G2ELib_V1/DC//AC Converters/Voltage Source Converters (VSC)/Grid-Forming VSC (GFM)/VSC - GFM - Generic - Ideal/Virtual Impedance ==
  Ig_dq0 : Inport
  Constant : Constant  Value=VI_Rv_pu
  Demux1 : Demux  Outputs=2
      settings: DisplayOption=none
  Gain1 : Gain  Gain=VI_Enable
  Gain5 : Gain  Gain=VI_Lv_pu/VI_Rv_pu
  Gain9 : Gain  Gain=VI_Lv_pu/VI_Rv_pu
  Mux2 : Mux  Inputs=3
  Selector : Selector  InputPortWidth=3  IndexOptions=Index vector (dialog)  Indices=[1 2]  OutputSizes=1
  Sum7 : Sum  Inputs=|+-
  Sum8 : Sum  Inputs=++|
  dEg_0 : Constant  Value=0
  product{,1..3} (4 alike) : Product  InputSameDT=on  RndMeth=Zero  SaturateOnIntegerOverflow=on  OutDataTypeStr=Inherit: Same as first input
  dEg_dq0_VI : Outport
  wires:
  Gain1/1 -> dEg_dq0_VI/1
  dEg_0/1 -> Mux2/3
  product3/1 -> Gain5/1
  Demux1/2 -> product3/1, product2/1  "igq"
  Mux2/1 -> Gain1/1
  Demux1/1 -> product/2, product1/1  "Igd"
  Gain9/1 -> Sum8/1
  Ig_dq0/1 -> Selector/1
  product2/1 -> Sum8/2
  product/1 -> Gain9/1
  Sum8/1 -> Mux2/2
  Gain5/1 -> Sum7/2
  Sum7/1 -> Mux2/1
  Selector/1 -> Demux1/1
  product1/1 -> Sum7/1
  Constant/1 -> product2/2, product1/2, product/1, product3/2
